simulink model "RobotControl"  (R2016a)
settings: Solver=FixedStepDiscrete  StartTime=0.0  StopTime=16  RelTol=1e-3
values from neighbouring files (symbols this model uses):
  BUSY = 16    [ControlInit.m]
  CLEANED = 18    [ControlInit.m]
  EMPTY = 17    [ControlInit.m]
  LEFT_BUSY_RIGHT_BUSY = 9    [ControlInit.m]
  LEFT_BUSY_RIGHT_CLEANED = 14    [ControlInit.m]
  LEFT_BUSY_RIGHT_EMPTY = 7    [ControlInit.m]
  LEFT_CLEANED_RIGHT_BUSY = 13    [ControlInit.m]
  LEFT_CLEANED_RIGHT_CLEANED = 12    [ControlInit.m]
  LEFT_CLEANED_RIGHT_EMPTY = 10    [ControlInit.m]
  LEFT_EMPTY_RIGHT_BUSY = 8    [ControlInit.m]
  LEFT_EMPTY_RIGHT_CLEANED = 11    [ControlInit.m]
  LEFT_EMPTY_RIGHT_EMPTY = 15    [ControlInit.m]
  ROB_EAST = 0    [ControlInit.m]
  ROB_NORTH = 270    [ControlInit.m]
  ROB_SOUTH = 90    [ControlInit.m]
  ROB_WEST = 180    [ControlInit.m]
  UNCOVERED = 19    [ControlInit.m]
settings Model: Creator=oelkawok  LastModifiedBy=omaro
settings DataIOCC: SaveOutput=off  SaveTime=off

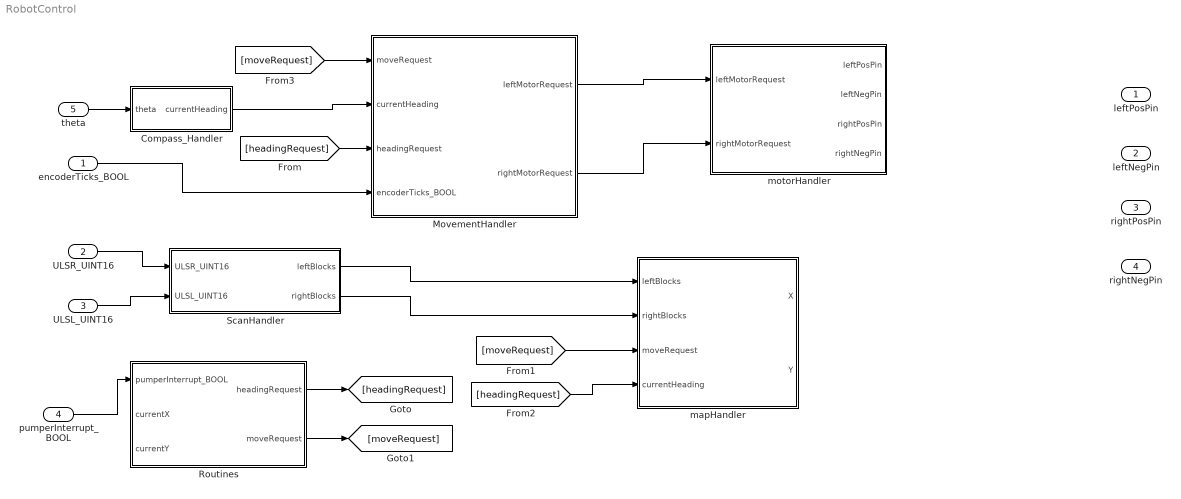
== system RobotControl ==
  encoderTicks_BOOL : Inport  OutDataTypeStr=boolean  PortDimensions=1  SampleTime=[0.0050000000000000001,0]
  ULSR_UINT16 : Inport  Port=2  OutDataTypeStr=uint16  PortDimensions=1  SampleTime=[0.0050000000000000001,0]
  ULSL_UINT16 : Inport  Port=3  OutDataTypeStr=uint16  PortDimensions=1  SampleTime=[0.0050000000000000001,0]
  pumperInterrupt_BOOL : Inport  Port=4  OutDataTypeStr=boolean  PortDimensions=1  SampleTime=[0.0050000000000000001,0]
  theta : Inport  Port=5  OutDataTypeStr=boolean  PortDimensions=1  SampleTime=[0.0050000000000000001,0]
  Compass_Handler : Subsystem
  MovementHandler : Subsystem
  Routines : Subsystem
  ScanHandler : Subsystem
  mapHandler : Subsystem
  motorHandler : Subsystem
  leftPosPin : Outport  OutDataTypeStr=double  PortDimensions=1
  leftNegPin : Outport  Port=2  OutDataTypeStr=double  PortDimensions=1
  rightPosPin : Outport  Port=3  OutDataTypeStr=double  PortDimensions=1
  rightNegPin : Outport  Port=4  OutDataTypeStr=double  PortDimensions=1
  wires:
  MovementHandler/1(leftMotorRequest) -> motorHandler/1(leftMotorRequest)
  MovementHandler/2(rightMotorRequest) -> motorHandler/2(rightMotorRequest)
  theta/1 -> Compass_Handler/1(theta)
  encoderTicks_BOOL/1 -> MovementHandler/4(encoderTicks_BOOL)
  Compass_Handler/1(currentHeading) -> MovementHandler/2(currentHeading)
  [headingRequest] -> MovementHandler/3(headingRequest)
  Routines/1(headingRequest) -> [headingRequest]
  Routines/2(moveRequest) -> [moveRequest]
  pumperInterrupt_BOOL/1 -> Routines/1(pumperInterrupt_BOOL)
  ULSL_UINT16/1 -> ScanHandler/2(ULSL_UINT16)
  ULSR_UINT16/1 -> ScanHandler/1(ULSR_UINT16)
  ScanHandler/1(leftBlocks) -> mapHandler/1(leftBlocks)
  ScanHandler/2(rightBlocks) -> mapHandler/2(rightBlocks)
  [moveRequest] -> mapHandler/3(moveRequest)
  [headingRequest] -> mapHandler/4(currentHeading)
  [moveRequest] -> MovementHandler/1(moveRequest)

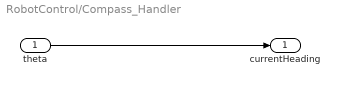
== system RobotControl/Compass_Handler ==
  theta : Inport
  currentHeading : Outport
  wires:
  theta/1 -> currentHeading/1

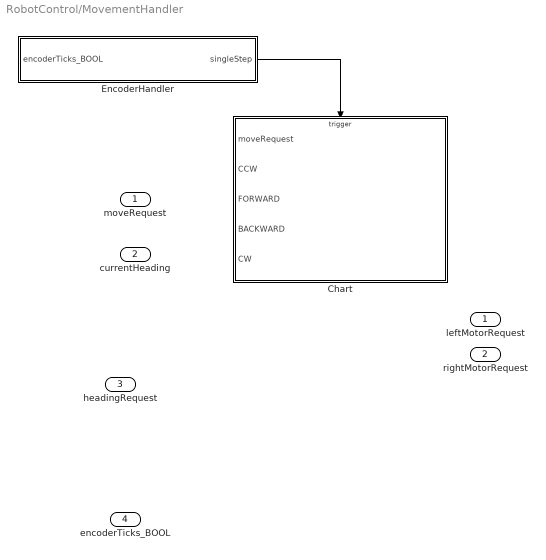
== system RobotControl/MovementHandler ==
  moveRequest : Inport
  currentHeading : Inport  Port=2
  headingRequest : Inport  Port=3
  encoderTicks_BOOL : Inport  Port=4  OutDataTypeStr=boolean  PortDimensions=1  SampleTime=[0.0050000000000000001,0]
  Chart : Stateflow chart  TreatAsAtomicUnit=on
  EncoderHandler : Subsystem
  leftMotorRequest : Outport
  rightMotorRequest : Outport  Port=2
  wires:
  EncoderHandler/1(singleStep) -> Chart/Trigger

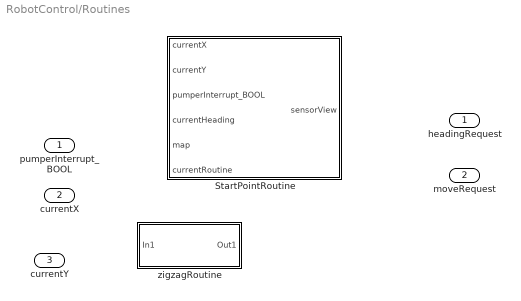
== system RobotControl/Routines ==
  pumperInterrupt_BOOL : Inport
  currentX : Inport  Port=2
  currentY : Inport  Port=3
  StartPointRoutine : Subsystem
  zigzagRoutine : Subsystem
  headingRequest : Outport
  moveRequest : Outport  Port=2

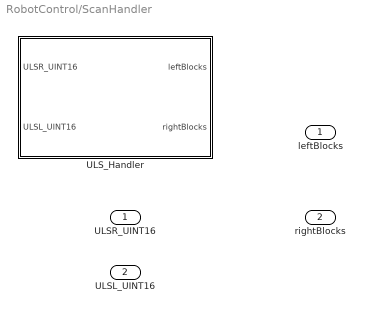
== system RobotControl/ScanHandler ==
  ULSR_UINT16 : Inport  OutDataTypeStr=uint16  PortDimensions=1  SampleTime=[0.0050000000000000001,0]
  ULSL_UINT16 : Inport  Port=2  OutDataTypeStr=uint16  PortDimensions=1  SampleTime=[0.0050000000000000001,0]
  ULS_Handler : Subsystem
  leftBlocks : Outport
  rightBlocks : Outport  Port=2

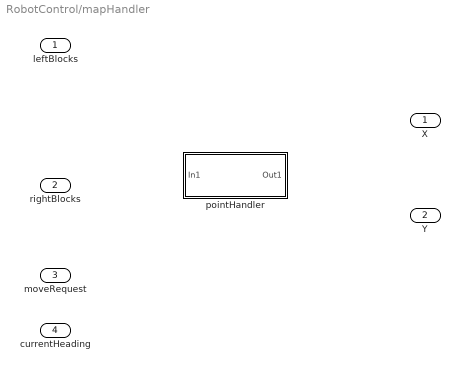
== system RobotControl/mapHandler ==
  leftBlocks : Inport
  rightBlocks : Inport  Port=2
  moveRequest : Inport  Port=3
  currentHeading : Inport  Port=4
  pointHandler : Subsystem
  X : Outport
  Y : Outport  Port=2

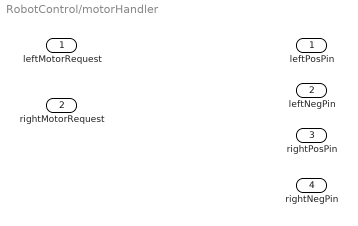
== system RobotControl/motorHandler ==
  leftMotorRequest : Inport
  rightMotorRequest : Inport  Port=2
  leftPosPin : Outport
  leftNegPin : Outport  Port=2
  rightPosPin : Outport  Port=3
  rightNegPin : Outport  Port=4

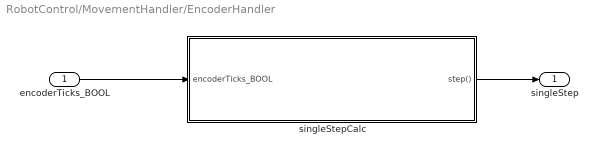
== system RobotControl/MovementHandler/EncoderHandler ==
  encoderTicks_BOOL : Inport  OutDataTypeStr=boolean  PortDimensions=1  SampleTime=[0.0050000000000000001,0]
  singleStepCalc : Stateflow chart  TreatAsAtomicUnit=on
  singleStep : Outport
  wires:
  encoderTicks_BOOL/1 -> singleStepCalc/1(encoderTicks_BOOL)
  singleStepCalc/1(step()) -> singleStep/1

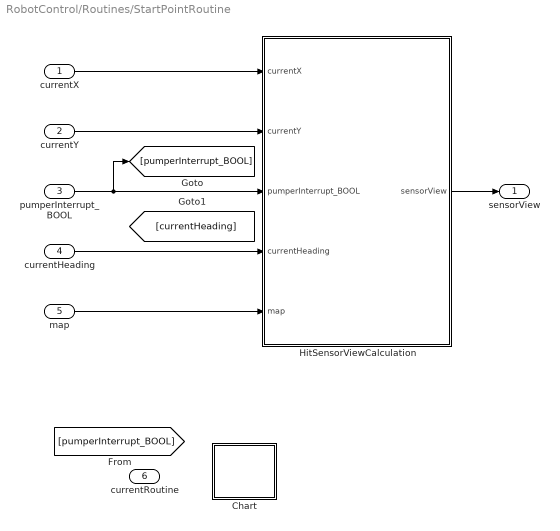
== system RobotControl/Routines/StartPointRoutine ==
  currentX : Inport
  currentY : Inport  Port=2
  pumperInterrupt_BOOL : Inport  Port=3
  currentHeading : Inport  Port=4
  map : Inport  Port=5
  currentRoutine : Inport  Port=6
  Chart : Stateflow chart  TreatAsAtomicUnit=on
  HitSensorViewCalculation : Subsystem
  sensorView : Outport
  wires:
  currentX/1 -> HitSensorViewCalculation/1(currentX)
  currentY/1 -> HitSensorViewCalculation/2(currentY)
  pumperInterrupt_BOOL/1 -> [pumperInterrupt_BOOL], HitSensorViewCalculation/3(pumperInterrupt_BOOL)
  currentHeading/1 -> HitSensorViewCalculation/4(currentHeading)
  map/1 -> HitSensorViewCalculation/5(map)
  HitSensorViewCalculation/1(sensorView) -> sensorView/1

== system RobotControl/Routines/zigzagRoutine ==
  In1 : Inport
  Out1 : Outport
  wires:
  In1/1 -> Out1/1

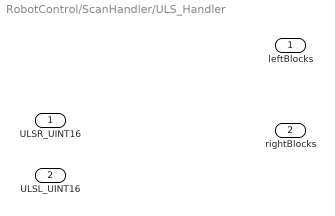
== system RobotControl/ScanHandler/ULS_Handler ==
  ULSR_UINT16 : Inport  OutDataTypeStr=uint16  PortDimensions=1  SampleTime=[0.0050000000000000001,0]
  ULSL_UINT16 : Inport  Port=2  OutDataTypeStr=uint16  PortDimensions=1  SampleTime=[0.0050000000000000001,0]
  leftBlocks : Outport
  rightBlocks : Outport  Port=2

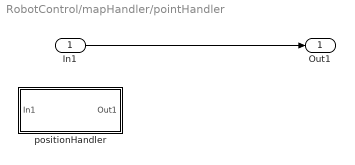
== system RobotControl/mapHandler/pointHandler ==
  In1 : Inport
  positionHandler : Subsystem
  Out1 : Outport
  wires:
  In1/1 -> Out1/1

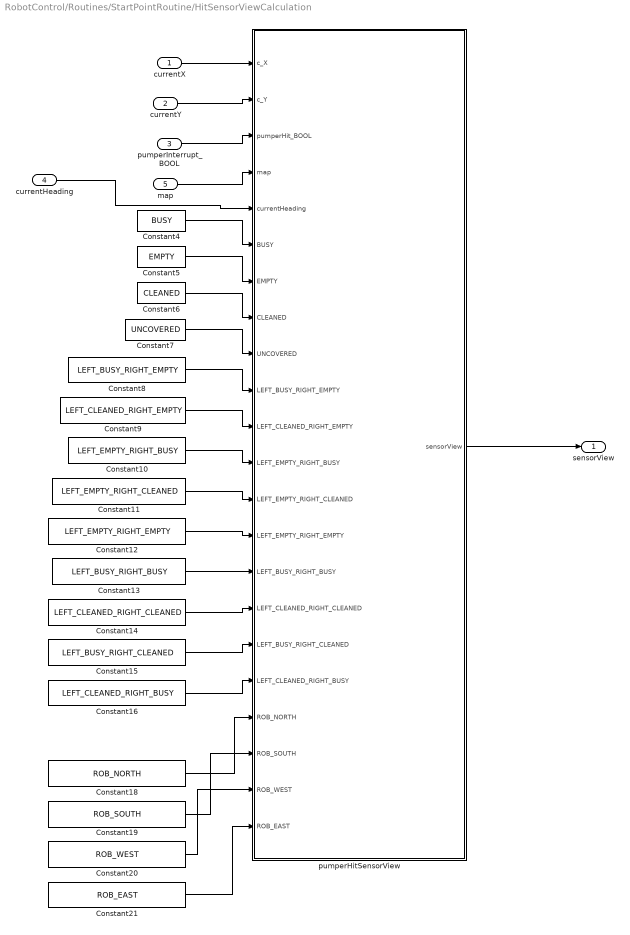
== system RobotControl/Routines/StartPointRoutine/HitSensorViewCalculation ==
  currentX : Inport
  currentY : Inport  Port=2
  pumperInterrupt_BOOL : Inport  Port=3
  currentHeading : Inport  Port=4
  map : Inport  Port=5
  Constant10 : Constant  Value=LEFT_EMPTY_RIGHT_BUSY
  Constant11 : Constant  Value=LEFT_EMPTY_RIGHT_CLEANED
  Constant12 : Constant  Value=LEFT_EMPTY_RIGHT_EMPTY
  Constant13 : Constant  Value=LEFT_BUSY_RIGHT_BUSY
  Constant14 : Constant  Value=LEFT_CLEANED_RIGHT_CLEANED
  Constant15 : Constant  Value=LEFT_BUSY_RIGHT_CLEANED
  Constant16 : Constant  Value=LEFT_CLEANED_RIGHT_BUSY
  Constant18 : Constant  Value=ROB_NORTH
  Constant19 : Constant  Value=ROB_SOUTH
  Constant20 : Constant  Value=ROB_WEST
  Constant21 : Constant  Value=ROB_EAST
  Constant4 : Constant  Value=BUSY
  Constant5 : Constant  Value=EMPTY
  Constant6 : Constant  Value=CLEANED
  Constant7 : Constant  Value=UNCOVERED
  Constant8 : Constant  Value=LEFT_BUSY_RIGHT_EMPTY
  Constant9 : Constant  Value=LEFT_CLEANED_RIGHT_EMPTY
  pumperHitSensorView : Stateflow chart  TreatAsAtomicUnit=on
  sensorView : Outport
  wires:
  Constant19/1 -> pumperHitSensorView/20(ROB_SOUTH)
  Constant21/1 -> pumperHitSensorView/22(ROB_EAST)
  Constant18/1 -> pumperHitSensorView/19(ROB_NORTH)
  Constant20/1 -> pumperHitSensorView/21(ROB_WEST)
  map/1 -> pumperHitSensorView/4(map)
  pumperInterrupt_BOOL/1 -> pumperHitSensorView/3(pumperHit_BOOL)
  currentX/1 -> pumperHitSensorView/1(c_X)
  currentY/1 -> pumperHitSensorView/2(c_Y)
  Constant8/1 -> pumperHitSensorView/10(LEFT_BUSY_RIGHT_EMPTY)
  Constant7/1 -> pumperHitSensorView/9(UNCOVERED)
  Constant5/1 -> pumperHitSensorView/7(EMPTY)
  Constant4/1 -> pumperHitSensorView/6(BUSY)
  Constant6/1 -> pumperHitSensorView/8(CLEANED)
  Constant10/1 -> pumperHitSensorView/12(LEFT_EMPTY_RIGHT_BUSY)
  Constant15/1 -> pumperHitSensorView/17(LEFT_BUSY_RIGHT_CLEANED)
  Constant12/1 -> pumperHitSensorView/14(LEFT_EMPTY_RIGHT_EMPTY)
  Constant13/1 -> pumperHitSensorView/15(LEFT_BUSY_RIGHT_BUSY)
  Constant9/1 -> pumperHitSensorView/11(LEFT_CLEANED_RIGHT_EMPTY)
  Constant11/1 -> pumperHitSensorView/13(LEFT_EMPTY_RIGHT_CLEANED)
  Constant14/1 -> pumperHitSensorView/16(LEFT_CLEANED_RIGHT_CLEANED)
  Constant16/1 -> pumperHitSensorView/18(LEFT_CLEANED_RIGHT_BUSY)
  pumperHitSensorView/1(sensorView) -> sensorView/1
  currentHeading/1 -> pumperHitSensorView/5(currentHeading)

== system RobotControl/mapHandler/pointHandler/positionHandler ==
  In1 : Inport
  Out1 : Outport
  wires:
  In1/1 -> Out1/1

== stateflow chart RobotControl/MovementHandler/Chart ==
  state forward
  state CW
  state backward
  state CCW
  (default) -> forward
  forward -> (junction 9)
  (junction 9) -> forward [order 1] : [moveRequest == FORWARD]
  (junction 9) -> backward [order 2] : [moveRequest == BACKWARD]
  CW -> (junction 9)
  backward -> (junction 9)
  (junction 9) -> CW [order 4] : [moveRequest == CW]
  CCW -> (junction 9)
  (junction 9) -> CCW [order 3] : [moveRequest == CCW]
  data: moveRequest input; CCW input; FORWARD input; BACKWARD input; CW input
  events: completeStep input FUNCTION_CALL_EVENT

== stateflow chart RobotControl/Routines/StartPointRoutine/HitSensorViewCalculation/pumperHitSensorView ==
  state SensorViewState
  state Init
    entry:
    sensorView = 0;
  state NoHit
    entry:
    currentY = c_Y - 1;
    currentX = c_X - 1;
  (junction 10) -> SensorViewState [order 1] : [(map[currentY][currentX - 1] == BUSY) ...
      | && ( (map[currentY][currentX + 1] == EMPTY)...
      |  || (map[currentY][currentX+1] == UNCOVERED) )]...
      | /sensorView = LEFT_BUSY_RIGHT_EMPTY;
  (junction 10) -> SensorViewState [order 2] : [(map[currentY][currentX - 1] == CLEANED) ...
      | && ((map[currentY][currentX + 1] == EMPTY)...
      | || (map[currentY][currentX+1] == UNCOVERED))]
      | /{sensorView =  LEFT_CLEANED_RIGHT_EMPTY;}
  (junction 10) -> SensorViewState [order 3] : [((map[currentY][currentX - 1] == EMPTY) ...
      | || (map[currentY][currentX - 1] == UNCOVERED))...
      | && (map[currentY][currentX + 1] == BUSY)]
      | /{sensorView = LEFT_EMPTY_RIGHT_BUSY;}
  (junction 10) -> SensorViewState [order 4] : [(map[currentY][currentX + 1] == CLEANED) ...
      | && ((map[currentY][currentX - 1] == EMPTY)...
      | || (map[currentY][currentX - 1] == UNCOVERED))]
      | /{sensorView =  LEFT_EMPTY_RIGHT_CLEANED;}
  (junction 10) -> SensorViewState [order 5] : [((map[currentY][currentX + 1] == EMPTY) ...
      | || (map[currentY][currentX + 1] == UNCOVERED))...
      | && ((map[currentY][currentX - 1] == EMPTY)...
      | || (map[currentY][currentX - 1] == UNCOVERED))]
      | /{sensorView = LEFT_EMPTY_RIGHT_EMPTY;}
  (junction 10) -> SensorViewState [order 6] : [(map[currentY][currentX - 1] == BUSY) ...
      | && (map[currentY][currentX + 1] == BUSY)]
      | /{sensorView = LEFT_BUSY_RIGHT_BUSY;}
  (junction 10) -> SensorViewState [order 7] : [(map[currentY][currentX - 1] == CLEANED) ...
      | && (map[currentY][currentX + 1] == CLEANED)]
      | /{sensorView = LEFT_CLEANED_RIGHT_CLEANED;}
  (junction 10) -> SensorViewState [order 8] : [(map[currentY][currentX - 1] == BUSY) ...
      | && (map[currentY][currentX + 1] == CLEANED)]
      | /{sensorView = LEFT_BUSY_RIGHT_CLEANED;}
  (junction 10) -> SensorViewState [order 9] : [(map[currentY][currentX - 1] == CLEANED) ...
      | && (map[currentY][currentX + 1] == BUSY)]
      | /{sensorView = LEFT_CLEANED_RIGHT_BUSY;}
  (junction 8) -> (junction 10) [order 1] : [currentHeading == ROB_NORTH]
  (default) -> Init
  (junction 11) -> SensorViewState [order 2] : [(map[currentY][currentX - 1] == BUSY) ...
      | && ( (map[currentY][currentX + 1] == EMPTY)...
      |  || (map[currentY][currentX+1] == UNCOVERED) )]...
      | /sensorView = LEFT_EMPTY_RIGHT_BUSY;
  Init -> NoHit
  NoHit -> (junction 8) : [pumperHit_BOOL]
  (junction 8) -> (junction 15) [order 4] : [currentHeading == ROB_EAST]
  (junction 8) -> (junction 13) [order 3] : [currentHeading == ROB_WEST]
  (junction 8) -> (junction 11) [order 2] : [currentHeading == ROB_SOUTH]
  SensorViewState -> NoHit
  (junction 11) -> SensorViewState [order 1] : [(map[currentY][currentX - 1] == CLEANED) ...
      | && ((map[currentY][currentX + 1] == EMPTY)...
      | || (map[currentY][currentX+1] == UNCOVERED))]
      | /{sensorView =  LEFT_EMPTY_RIGHT_CLEANED;}
  (junction 11) -> SensorViewState [order 5] : [((map[currentY][currentX - 1] == EMPTY) ...
      | || (map[currentY][currentX - 1] == UNCOVERED))...
      | && (map[currentY][currentX + 1] == BUSY)]
      | /{sensorView = LEFT_BUSY_RIGHT_EMPTY;}
  (junction 11) -> SensorViewState [order 6] : [(map[currentY][currentX + 1] == CLEANED) ...
      | && ((map[currentY][currentX - 1] == EMPTY)...
      | || (map[currentY][currentX - 1] == UNCOVERED))]
      | /{sensorView =  LEFT_CLEANED_RIGHT_EMPTY;}
  (junction 11) -> SensorViewState [order 4] : [((map[currentY][currentX + 1] == EMPTY) ...
      | || (map[currentY][currentX + 1] == UNCOVERED))...
      | && ((map[currentY][currentX - 1] == EMPTY)...
      | || (map[currentY][currentX - 1] == UNCOVERED))]
      | /{sensorView = LEFT_EMPTY_RIGHT_EMPTY;}
  (junction 11) -> SensorViewState [order 8] : [(map[currentY][currentX - 1] == BUSY) ...
      | && (map[currentY][currentX + 1] == CLEANED)]
      | /{sensorView = LEFT_CLEANED_RIGHT_BUSY;}
  (junction 11) -> SensorViewState [order 3] : [(map[currentY][currentX - 1] == BUSY) ...
      | && (map[currentY][currentX + 1] == BUSY)]
      | /{sensorView = LEFT_BUSY_RIGHT_BUSY;}
  (junction 11) -> SensorViewState [order 7] : [(map[currentY][currentX - 1] == CLEANED) ...
      | && (map[currentY][currentX + 1] == CLEANED)]
      | /{sensorView = LEFT_CLEANED_RIGHT_CLEANED;}
  (junction 11) -> SensorViewState [order 9] : [(map[currentY][currentX - 1] == CLEANED) ...
      | && (map[currentY][currentX + 1] == BUSY)]
      | /{sensorView = LEFT_BUSY_RIGHT_CLEANED;}
  data: c_X input; c_Y input; pumperHit_BOOL input; sensorView output uint8; map input size=[19 19]; currentHeading input; BUSY input; EMPTY input; CLEANED input; UNCOVERED input; LEFT_BUSY_RIGHT_EMPTY input; LEFT_CLEANED_RIGHT_EMPTY input; LEFT_EMPTY_RIGHT_BUSY input; LEFT_EMPTY_RIGHT_CLEANED input; LEFT_EMPTY_RIGHT_EMPTY input; LEFT_BUSY_RIGHT_BUSY input; LEFT_CLEANED_RIGHT_CLEANED input; LEFT_BUSY_RIGHT_CLEANED input; LEFT_CLEANED_RIGHT_BUSY input; ROB_NORTH input; ROB_SOUTH input; ROB_WEST input; ROB_EAST input; currentX local uint8; currentY local uint8

== stateflow chart RobotControl/MovementHandler/EncoderHandler/singleStepCalc ==
  state Init
    entry:
    counter = 0;
  state High
  state Low
    entry:
    counter++;
  state step
    entry:
    step;
    counter = 0;
  (default) -> Init
  High -> Low : [encoderTicks_BOOL < 1000]
  Init -> High
  Low -> High [order 1] : [encoderTicks_BOOL> 1000]
  step -> High
  Low -> step [order 2] : [counter >= 30]
  data: encoderTicks_BOOL input; counter local uint8
  events: step output FUNCTION_CALL_EVENT

== stateflow chart RobotControl/Routines/StartPointRoutine/Chart ==
